simulink model "balanceCAOv1"  (R2019b)
settings: Solver=VariableStepAuto  StartTime=0.0  StopTime=6.5  RelTol=1e-3
model workspace (MAT data in the model file):
  F = [0 0 0 0 0 0 0 0 0 0 0 0 0 0 0 0 0 0 0 0 0]
  K = 1
  a1 = 0.000261007117673
  b1 = 0.618793924538
  c1 = 77.6367098126
  coeffs = [11319432.2907 569821497 46409.5443403 1.75479262565e-09]
  dt = 2e-05
  dx = 0.0133333333333
  nx = 21
  t1 = 1
  t2 = 1
  th = 1
  w = [0 0 0 0 0 0 0 0 0 0 0 0 0 0 0 0 0 0 0 0 0]
  w_init = [1 2 3 4 5 6 7 8 9 10 11 12 13 14 15 16 17 18 19 20 21]
  w_new = [0 0 0 0 0 0 0 0 0 0 0 0 0 0 0 0 0 0 0 0 0]
  w_old = [0 0 0 0 0 0 0 0 0 0 0 0 0 0 0 0 0 0 0 0 0]
values from neighbouring files (symbols this model uses):
  B = 0.033125    [Lame_worspace.mat]    (also in Launcher.m = 0.928190886807; Parameters.mat = 0.441493924538; Poutre_diff.m = 0.441493924538; Workspace_lame.mat = 0.441493924538)
  f = 12.17    [Launcher.m]    (also in Parameters.mat; Poutre_diff.m; Workspace_lame.mat)
  J = 2.732709375e-11    [Lame_worspace.mat]    (also in Launcher.m = 2.47880205e-11; Parameters.mat = 2.47880205e-11; Poutre_diff.m = 2.47880205e-11; Workspace_lame.mat = 2.47880205e-11)
  L = 0.24    [Lame_worspace.mat]    (also in Launcher.m; Parameters.mat; Poutre_diff.m; Workspace_lame.mat)
undefined symbols (not defined in the file or in its folder): aO, D, dE, eL, Kamp, Kc, kd, Ke, ki, kp, masse, mLame, N, R, R1, R2, R3, R4, Req, to, Vd1, Vd2, Voffset
settings Model: Creator=lucas  LastModifiedBy=lucas

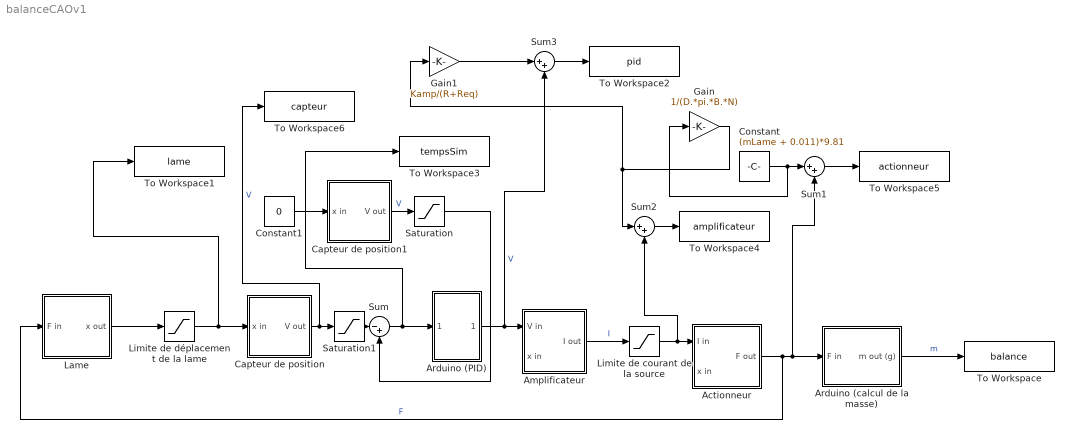
== system balanceCAOv1 ==
  Actionneur : Subsystem
  Amplificateur : Subsystem
  Arduino (PID) : Subsystem
  Arduino (calcul de la masse) : Subsystem
  Capteur de position : Subsystem
  Capteur de position1 : Subsystem
  Constant : Constant  Value=(mLame + 0.011)*9.81  SampleTime=dt
  Constant1 : Constant  Value=0  SampleTime=dt
  Gain : Gain  Gain=1/(D.*pi.*B.*N)
  Gain1 : Gain  Gain=Kamp/(R+Req)
  Lame : Subsystem
  Limite de courant de la source : Saturate  UpperLimit=3  LowerLimit=-inf
  Limite de déplacement de la lame : Saturate  UpperLimit=(dE-eL)/2  LowerLimit=-(dE-eL)/2
  Saturation : Saturate  UpperLimit=5  LowerLimit=0
  Saturation1 : Saturate  UpperLimit=5  LowerLimit=0
  Sum : Sum  Inputs=|-+
  Sum1 : Sum  Inputs=|++
  Sum2 : Sum  Inputs=|++
  Sum3 : Sum  Inputs=|++
  To Workspace : ToWorkspace  VariableName=balance  SaveFormat=Timeseries  SampleTime=1/9600
  To Workspace1 : ToWorkspace  VariableName=lame  SaveFormat=Timeseries  SampleTime=1/9600
  To Workspace2 : ToWorkspace  VariableName=pid  SaveFormat=Timeseries  SampleTime=1/9600
  To Workspace3 : ToWorkspace  VariableName=tempsSim  SaveFormat=Timeseries  SampleTime=1/9600
  To Workspace4 : ToWorkspace  VariableName=amplificateur  SaveFormat=Timeseries  SampleTime=1/9600
  To Workspace5 : ToWorkspace  VariableName=actionneur  SaveFormat=Timeseries  SampleTime=1/9600
  To Workspace6 : ToWorkspace  VariableName=capteur  SaveFormat=Timeseries  SampleTime=1/9600
  wires:
  Actionneur/1(F out) -> Sum1/2, Arduino (calcul de la masse)/1(F in), Lame/1(F in)  "F"
  Arduino (calcul de la masse)/1(m out (g)) -> To Workspace/1  "m"
  Arduino (PID)/1(V out) -> Sum3/2, Amplificateur/1(V in)  "V"
  Sum/1 -> To Workspace3/1, Arduino (PID)/1(V in)
  Constant1/1 -> Capteur de position1/1(x in)
  Lame/1(x out) -> Limite de déplacement de la lame/1
  Amplificateur/1(I out) -> Limite de courant de la source/1  "I"
  Limite de courant de la source/1 -> Sum2/2, Actionneur/1(I in)
  Capteur de position1/1(V out) -> Saturation/1  "V"
  Saturation/1 -> Sum/2
  Capteur de position/1(V out) -> To Workspace6/1, Saturation1/1  "V"
  Saturation1/1 -> Sum/1
  Sum1/1 -> To Workspace5/1
  Constant/1 -> Gain/1, Sum1/1
  Sum2/1 -> To Workspace4/1
  Gain/1 -> Sum2/1, Gain1/1
  Gain1/1 -> Sum3/1
  Sum3/1 -> To Workspace2/1
  Limite de déplacement de la lame/1 -> To Workspace1/1, Capteur de position/1(x in)

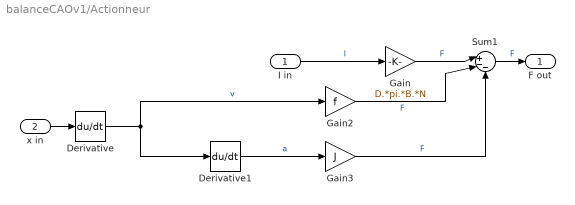
== system balanceCAOv1/Actionneur ==
  I in : Inport
  x in : Inport  Port=2
  Derivative : Derivative
  Derivative1 : Derivative
  Gain : Gain  Gain=D.*pi.*B.*N
  Gain2 : Gain  Gain=f
  Gain3 : Gain  Gain=J
  Sum1 : Sum  Inputs=|+--
  F out : Outport
  wires:
  I in/1 -> Gain/1  "I"
  Gain/1 -> Sum1/1  "F"
  Derivative/1 -> Derivative1/1, Gain2/1  "v"
  x in/1 -> Derivative/1
  Gain2/1 -> Sum1/2  "F"
  Derivative1/1 -> Gain3/1  "a"
  Gain3/1 -> Sum1/3  "F"
  Sum1/1 -> F out/1  "F"

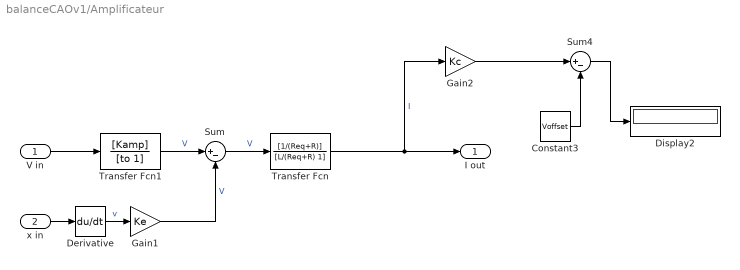
== system balanceCAOv1/Amplificateur ==
  V in : Inport
  x in : Inport  Port=2
  Constant3 : Constant  Value=Voffset  SampleTime=dt
  Derivative : Derivative
  Display2 : Display
  Gain1 : Gain  Gain=Ke
  Gain2 : Gain  Gain=Kc
  Sum : Sum  Inputs=|+-
  Sum4 : Sum  Inputs=|+-
  Transfer Fcn : TransferFcn  Numerator=[1/(Req+R)]  Denominator=[L/(Req+R) 1]
  Transfer Fcn1 : TransferFcn  Numerator=[Kamp]  Denominator=[to 1]
  I out : Outport
  wires:
  V in/1 -> Transfer Fcn1/1
  x in/1 -> Derivative/1
  Derivative/1 -> Gain1/1  "v"
  Gain1/1 -> Sum/2  "V"
  Sum/1 -> Transfer Fcn/1  "V"
  Transfer Fcn/1 -> I out/1, Gain2/1  "I"
  Transfer Fcn1/1 -> Sum/1  "V"
  Constant3/1 -> Sum4/2
  Gain2/1 -> Sum4/1
  Sum4/1 -> Display2/1

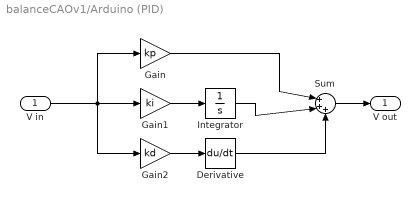
== system balanceCAOv1/Arduino (PID) ==
  V in : Inport
  Derivative : Derivative
  Gain : Gain  Gain=kp
  Gain1 : Gain  Gain=ki
  Gain2 : Gain  Gain=kd
  Integrator : Integrator
  Sum : Sum  Inputs=|+++
  V out : Outport
  wires:
  Derivative/1 -> Sum/3
  Integrator/1 -> Sum/2
  Gain/1 -> Sum/1
  Sum/1 -> V out/1
  V in/1 -> Gain2/1, Gain1/1, Gain/1
  Gain2/1 -> Derivative/1
  Gain1/1 -> Integrator/1

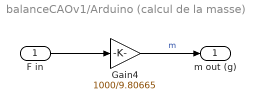
== system balanceCAOv1/Arduino (calcul de la masse) ==
  F in : Inport
  Gain4 : Gain  Gain=1000/9.80665
  m out (g) : Outport
  wires:
  Gain4/1 -> m out (g)/1  "m"
  F in/1 -> Gain4/1

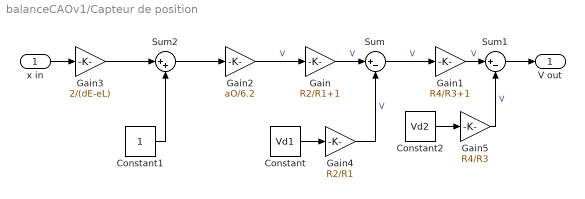
== system balanceCAOv1/Capteur de position ==
  x in : Inport
  Constant : Constant  Value=Vd1  SampleTime=dt
  Constant1 : Constant  SampleTime=dt
  Constant2 : Constant  Value=Vd2  SampleTime=dt
  Gain : Gain  Gain=R2/R1+1
  Gain1 : Gain  Gain=R4/R3+1
  Gain2 : Gain  Gain=aO/6.2
  Gain3 : Gain  Gain=2/(dE-eL)
  Gain4 : Gain  Gain=R2/R1
  Gain5 : Gain  Gain=R4/R3
  Sum : Sum  Inputs=|+-
  Sum1 : Sum  Inputs=|+-
  Sum2 : Sum  Inputs=|++
  V out : Outport
  wires:
  Constant1/1 -> Sum2/2
  x in/1 -> Gain3/1
  Gain3/1 -> Sum2/1
  Sum2/1 -> Gain2/1
  Gain2/1 -> Gain/1  "V"
  Gain/1 -> Sum/1  "V"
  Gain1/1 -> Sum1/1  "V"
  Sum1/1 -> V out/1
  Constant/1 -> Gain4/1
  Gain4/1 -> Sum/2  "V"
  Constant2/1 -> Gain5/1
  Gain5/1 -> Sum1/2  "V"
  Sum/1 -> Gain1/1  "V"

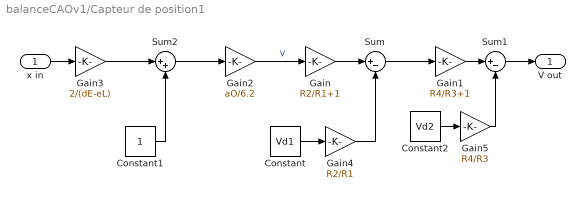
== system balanceCAOv1/Capteur de position1 ==
  x in : Inport
  Constant : Constant  Value=Vd1  SampleTime=dt
  Constant1 : Constant  SampleTime=dt
  Constant2 : Constant  Value=Vd2  SampleTime=dt
  Gain : Gain  Gain=R2/R1+1
  Gain1 : Gain  Gain=R4/R3+1
  Gain2 : Gain  Gain=aO/6.2
  Gain3 : Gain  Gain=2/(dE-eL)
  Gain4 : Gain  Gain=R2/R1
  Gain5 : Gain  Gain=R4/R3
  Sum : Sum  Inputs=|+-
  Sum1 : Sum  Inputs=|+-
  Sum2 : Sum  Inputs=|++
  V out : Outport
  wires:
  Constant1/1 -> Sum2/2
  x in/1 -> Gain3/1
  Gain3/1 -> Sum2/1
  Sum2/1 -> Gain2/1
  Gain2/1 -> Gain/1  "V"
  Gain/1 -> Sum/1
  Gain1/1 -> Sum1/1
  Sum1/1 -> V out/1
  Constant/1 -> Gain4/1
  Gain4/1 -> Sum/2
  Constant2/1 -> Gain5/1
  Gain5/1 -> Sum1/2
  Sum/1 -> Gain1/1

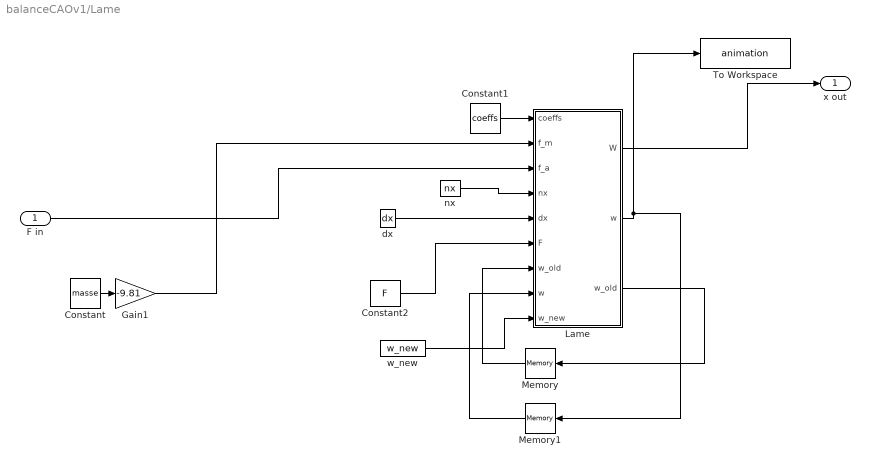
== system balanceCAOv1/Lame ==
  F in : Inport
  Constant : Constant  Value=masse  SampleTime=dt
  Constant1 : Constant  Value=coeffs  SampleTime=dt
  Constant2 : Constant  Value=F  SampleTime=dt
  Gain1 : Gain  Gain=-9.81
  Lame : MATLAB Function  TreatAsAtomicUnit=on
  Memory : Memory  InitialCondition=zeros(1,nx)
  Memory1 : Memory  InitialCondition=zeros(1,nx)
  To Workspace : ToWorkspace  VariableName=animation  SaveFormat=Timeseries  SampleTime=1/100
  dx : Constant  Value=dx  SampleTime=dt
  nx : Constant  Value=nx  SampleTime=dt
  w_new : Constant  Value=w_new  SampleTime=dt
  x out : Outport
  wires:
  F in/1 -> Lame/3(f_a)
  Memory1/1 -> Lame/8("w ")
  Constant2/1 -> Lame/6(F)
  Constant1/1 -> Lame/1(coeffs)
  w_new/1 -> Lame/9(w_new)
  nx/1 -> Lame/4(nx)
  dx/1 -> Lame/5(dx)
  Lame/1(W) -> x out/1
  Lame/2(w) -> To Workspace/1, Memory1/1
  Constant/1 -> Gain1/1
  Lame/3(w_old) -> Memory/1
  Memory/1 -> Lame/7("w_old ")
  Gain1/1 -> Lame/2(f_m)

== matlab function balanceCAOv1/Lame/Lame ==
  data: coeffs input; f_m input; W output; f_a input; nx input; dx input; F input; w_old input; w input; w_new input; w output; w_old output
function [W, w, w_old] = fcn(coeffs, f_m, f_a, nx, dx, F, w_old, w, w_new) 
     
    % La force
    F(round(nx/2)) = f_a + f_m;

    for i = 3:nx-2
        
        %Équation différentielle résolue par Sam
        w_new(i) = (-coeffs(1)*(w(i+2)-4*w(i+1)+6*w(i)-4*w(i-1)+w(i-2)) - coeffs(2)*(-2*w(i)+w_old(i)) + coeffs(3)*w(i) + F(i)/dx)*coeffs(4);

        %% Conditions limites 
        w_new(1:2) =0;                                 % Clampé à zero, position et dérivée nulle (le bout de la lame est fixe)
        w_new(end-1) = 2*w_new(end-2)-w_new(end-3);    % Libre au bout, dérivées 2e et 3e nulles
        w_new(end) = 2*w_new(end-1)-w_new(end-2);
       
    end
     
    %% Préparation du prochain tour
    
    w_old = w;
    w = w_new;
    W = w(end);
end
